simulink model "open_loop_dyn"  (R2022a)
settings: Solver=FixedStepAuto  StartTime=0.0  StopTime=10.0  FixedStep=0.01  RelTol=1e-3
undefined symbols (not defined in the file): dt, f, fx, fy, fz, nx, ny, nz, tau
settings Model: Creator=charl  LastModifiedBy=charl

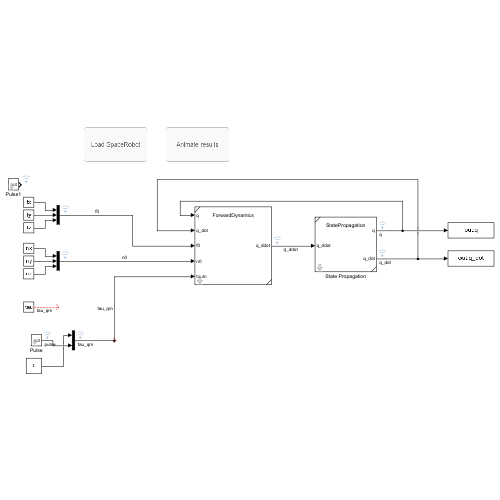
[thumbnail: Simulink's stored preview of the top-level diagram]
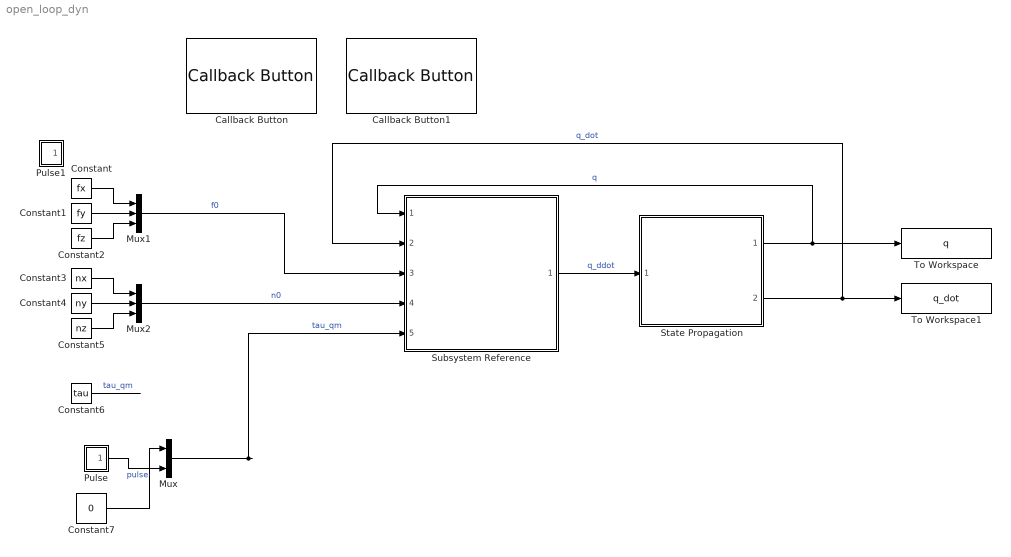
== system open_loop_dyn ==
  Callback Button : CallbackButton  ButtonText=Load SpaceRobot
      settings: ClickFcn=|
      | load('SC_2DoF.mat')
      | sc.homeConfig;
  Callback Button1 : CallbackButton  ButtonText=Animate results
      settings: ClickFcn=|
      | close all
      | sr.animate(out.q, 'fps', 17, 'rate', 1);
  Constant : Constant  Value=fx
  Constant1 : Constant  Value=fy
  Constant2 : Constant  Value=fz
  Constant3 : Constant  Value=nx
  Constant4 : Constant  Value=ny
  Constant5 : Constant  Value=nz
  Constant6 : Constant  Value=tau
  Constant7 : Constant  Value=0
  Mux : Mux  Inputs=2
  Mux1 : Mux  Inputs=3
  Mux2 : Mux  Inputs=3
  Pulse : Subsystem  mask{t_start=1, f=f, dt=dt}
      mask prompts: t_start "Start Time"; f "Amplitude"; dt "Width"
  Pulse1 : Subsystem  mask{t_start=1, f=f, dt=dt}
      mask prompts: t_start "Start Time"; f "Amplitude"; dt "Width"
  State Propagation : Subsystem  ReferencedSubsystem=StatePropagation  spaceRobot=sr  q_0=q_0  q_dot_0=q_dot_0
  Subsystem Reference : Subsystem  ReferencedSubsystem=ForwardDynamics  spaceRobot=sr  SimulateUsing=Interpreted execution
  To Workspace : ToWorkspace  VariableName=q  SaveFormat=Timeseries  SampleTime=-1
  To Workspace1 : ToWorkspace  VariableName=q_dot  SaveFormat=Timeseries  SampleTime=-1
  wires:
  Subsystem Reference/1 -> State Propagation/1  "q_ddot"
  Mux2/1 -> Subsystem Reference/4  "n0"
  State Propagation/1 -> Subsystem Reference/1, To Workspace/1  "q"
  State Propagation/2 -> Subsystem Reference/2, To Workspace1/1  "q_dot"
  Mux1/1 -> Subsystem Reference/3  "f0"
  Constant1/1 -> Mux1/2
  Constant2/1 -> Mux1/3
  Constant4/1 -> Mux2/2
  Constant3/1 -> Mux2/1
  Constant5/1 -> Mux2/3
  Pulse/1(out) -> Mux/2  "pulse"
  Constant7/1 -> Mux/1
  Constant/1 -> Mux1/1
  Mux/1 -> Subsystem Reference/5  "tau_qm"
  Constant6/1 -> ?  "tau_qm"

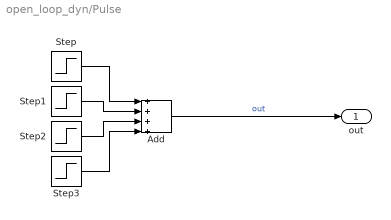
== system open_loop_dyn/Pulse ==
  Add : Sum  Inputs=++++
  Step : Step  Time=t_start  After=f  SampleTime=0
  Step1 : Step  Time=t_start+dt  After=-f  SampleTime=0
  Step2 : Step  Time=t_start+2*dt  After=-f  SampleTime=0
  Step3 : Step  Time=t_start+3*dt  After=f  SampleTime=0
  out : Outport
  wires:
  Step3/1 -> Add/4
  Add/1 -> out/1  "out"
  Step2/1 -> Add/3
  Step1/1 -> Add/2
  Step/1 -> Add/1

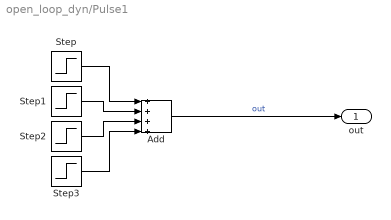
== system open_loop_dyn/Pulse1 ==
  Add : Sum  Inputs=++++
  Step : Step  Time=t_start  After=f  SampleTime=0
  Step1 : Step  Time=t_start+dt  After=-f  SampleTime=0
  Step2 : Step  Time=t_start+2*dt  After=-f  SampleTime=0
  Step3 : Step  Time=t_start+3*dt  After=f  SampleTime=0
  out : Outport
  wires:
  Step3/1 -> Add/4
  Add/1 -> out/1  "out"
  Step2/1 -> Add/3
  Step1/1 -> Add/2
  Step/1 -> Add/1
